simulink model "flightControlSystem"  (R2024b)
settings: Solver=ode3  StartTime=0  StopTime=10  FixedStep=Ts  RelTol=1e-3  EnableMultiTasking=on
undefined symbols (not defined in the file): codertarget, Controller, DiscIntNeverNeededParam, Discrete, Estimator, g, init, Sensors, Time, Ts, var_acc_angle_N, var_bias_gyr_N, var_gyro_p_N, Vehicle
libraries: simulink x39, sharedtransform x8, slpidlib x4, ctrlSharedLib x4, parrotlib x1
(part 3 of 3)

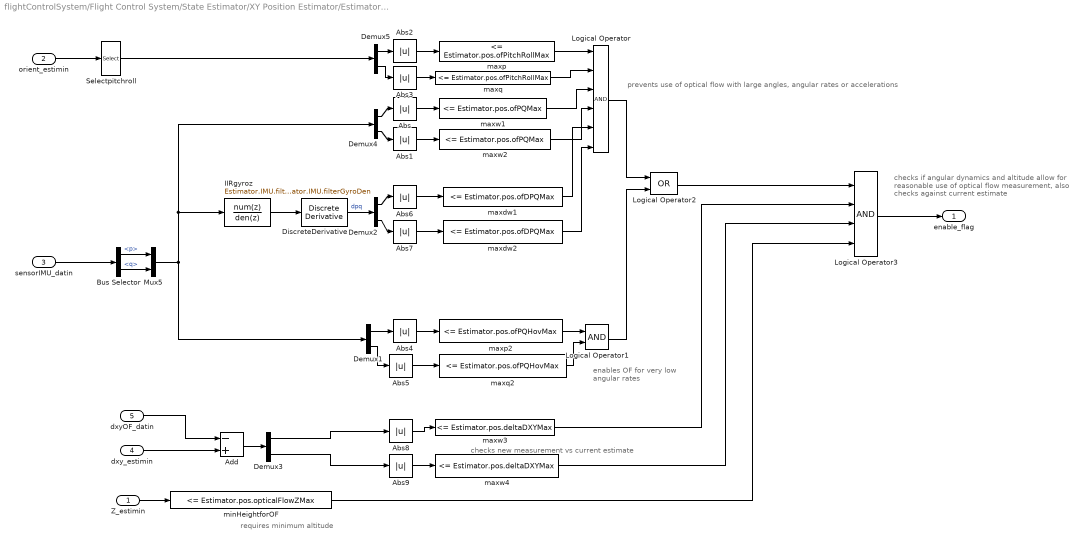
== system flightControlSystem/Flight Control System/State Estimator/XY Position Estimator/EstimatorVelocity/DataHandling ==
  note: prevents use of optical flow with large angles, angular rates or accelerations
  note: enables OF for very
      | low angular rates
  note: checks if angular dynamics and altitude allow for
      | reasonable use of optical flow measurement,
      | also checks against current estimate
  note: checks new measurement vs current estimate
  note: requires minimum altitude
  Z_estimin : Inport
  orient_estimin : Inport  Port=2
  sensorIMU_datin : Inport  Port=3
  dxy_estimin : Inport  Port=4
  dxyOF_datin : Inport  Port=5
  Abs{,1..9} (10 alike) : Abs  SaturateOnIntegerOverflow=off
  Add : Sum  Inputs=-+
  Bus Selector : BusSelector  OutputSignals=p,q
  Demux{1..5} (5 alike) : Demux  Outputs=2
  DiscreteDerivative : simulink/Discrete/Discrete Derivative  gainval=1.0  ICPrevScaledInput=0.0  OutMin=[]  OutMax=[]  OutDataType=fixdt(1, 16)  OutScaling=2^-10  DoSatur=off
  IIRgyroz : DiscreteFilter  Numerator=Estimator.IMU.filterGyroNum  Denominator=Estimator.IMU.filterGyroDen
  Logical Operator : Logic  Inputs=6  AllPortsSameDT=off  OutDataTypeStr=boolean
  Logical Operator1 : Logic  AllPortsSameDT=off  OutDataTypeStr=boolean
  Logical Operator2 : Logic  Operator=OR  AllPortsSameDT=off  OutDataTypeStr=boolean
  Logical Operator3 : Logic  Inputs=4  AllPortsSameDT=off  OutDataTypeStr=boolean
  Mux5 : Mux  Inputs=2
  Selectpitchroll : Selector  InputPortWidth=3  IndexOptions=Index vector (dialog)  Indices=[2 3]  OutputSizes=1
  maxdw1 : simulink/Logic and Bit Operations/Compare To Constant  relop=<=  const=Estimator.pos.ofDPQMax  OutDataTypeStr=boolean
  maxdw2 : simulink/Logic and Bit Operations/Compare To Constant  relop=<=  const=Estimator.pos.ofDPQMax  OutDataTypeStr=boolean
  maxp : simulink/Logic and Bit Operations/Compare To Constant  relop=<=  const=Estimator.pos.ofPitchRollMax  OutDataTypeStr=boolean
  maxp2 : simulink/Logic and Bit Operations/Compare To Constant  relop=<=  const=Estimator.pos.ofPQHovMax  OutDataTypeStr=boolean
  maxq : simulink/Logic and Bit Operations/Compare To Constant  relop=<=  const=Estimator.pos.ofPitchRollMax  OutDataTypeStr=boolean
  maxq2 : simulink/Logic and Bit Operations/Compare To Constant  relop=<=  const=Estimator.pos.ofPQHovMax  OutDataTypeStr=boolean
  maxw1 : simulink/Logic and Bit Operations/Compare To Constant  relop=<=  const=Estimator.pos.ofPQMax  OutDataTypeStr=boolean
  maxw2 : simulink/Logic and Bit Operations/Compare To Constant  relop=<=  const=Estimator.pos.ofPQMax  OutDataTypeStr=boolean
  maxw3 : simulink/Logic and Bit Operations/Compare To Constant  relop=<=  const=Estimator.pos.deltaDXYMax  OutDataTypeStr=boolean
  maxw4 : simulink/Logic and Bit Operations/Compare To Constant  relop=<=  const=Estimator.pos.deltaDXYMax  OutDataTypeStr=boolean
  minHeightforOF : simulink/Logic and Bit Operations/Compare To Constant  relop=<=  const=Estimator.pos.opticalFlowZMax  OutDataTypeStr=boolean
  enable_flag : Outport  VectorParamsAs1DForOutWhenUnconnected=off
  wires:
  minHeightforOF/1 -> Logical Operator3/4
  IIRgyroz/1 -> DiscreteDerivative/1
  Mux5/1 -> Demux1/1, Demux4/1, IIRgyroz/1
  maxw4/1 -> Logical Operator3/3
  maxw3/1 -> Logical Operator3/2
  dxyOF_datin/1 -> Add/1
  Demux3/2 -> Abs9/1
  Demux3/1 -> Abs8/1
  dxy_estimin/1 -> Add/2
  Add/1 -> Demux3/1
  Abs9/1 -> maxw4/1
  Abs8/1 -> maxw3/1
  Logical Operator2/1 -> Logical Operator3/1
  Logical Operator3/1 -> enable_flag/1
  DiscreteDerivative/1 -> Demux2/1  "dpq"
  Demux2/2 -> Abs7/1
  Demux2/1 -> Abs6/1
  Abs7/1 -> maxdw2/1
  Abs6/1 -> maxdw1/1
  Logical Operator1/1 -> Logical Operator2/2
  Demux1/2 -> Abs5/1
  Demux1/1 -> Abs4/1
  Abs5/1 -> maxq2/1
  Abs4/1 -> maxp2/1
  Abs3/1 -> maxq/1
  Abs2/1 -> maxp/1
  Demux4/2 -> Abs1/1
  Demux4/1 -> Abs/1
  Abs1/1 -> maxw2/1
  Abs/1 -> maxw1/1
  Z_estimin/1 -> minHeightforOF/1
  Logical Operator/1 -> Logical Operator2/1
  maxw1/1 -> Logical Operator/3
  Bus Selector/1 -> Mux5/1  "<p>"
  Selectpitchroll/1 -> Demux5/1
  sensorIMU_datin/1 -> Bus Selector/1
  maxq2/1 -> Logical Operator1/2
  Bus Selector/2 -> Mux5/2  "<q>"
  maxp/1 -> Logical Operator/1
  maxw2/1 -> Logical Operator/4
  orient_estimin/1 -> Selectpitchroll/1
  maxdw1/1 -> Logical Operator/5
  maxdw2/1 -> Logical Operator/6
  maxq/1 -> Logical Operator/2
  Demux5/1 -> Abs2/1
  Demux5/2 -> Abs3/1
  maxp2/1 -> Logical Operator1/1

== system flightControlSystem/Flight Control System/State Estimator/XY Position Estimator/EstimatorVelocity/XY velocity w//o angular velocity compensation ==
  note: Optical flow raw readings are converted to velocity in m/s based on the estimated altitude
  optical_flow : Inport
  z_estimate : Inport  Port=2
  " " : Product  Inputs=**
  Compare To Constant : simulink/Logic and Bit Operations/Compare To Constant  relop=<  const=200*4  OutDataTypeStr=boolean
  Counter Free-Running : simulink/Sources/Counter Free-Running  NumBits=32  tsamp=-1
  Gain : Gain  Gain=-1
  Select dxy : Selector  InputPortWidth=3  IndexOptions=Index vector (dialog)  Indices=[1 2]  OutputSizes=1
  Switch : Switch  Criteria=u2 > Threshold  SaturateOnIntegerOverflow=off  InputSameDT=off
  opticalFlowErrorCorrect : Gain  Gain=1.15
  optical_flow_dx_dy : Outport
  wires:
  Select dxy/1 -> optical_flow_dx_dy/1  "optical_flow_dx_dy"
  " "/1 -> opticalFlowErrorCorrect/1
  opticalFlowErrorCorrect/1 -> Switch/3
  Gain/1 -> " "/2
  Switch/1 -> Select dxy/1
  Counter Free-Running/1 -> Compare To Constant/1
  Compare To Constant/1 -> Switch/2
  optical_flow/1 -> " "/1, Switch/1
  z_estimate/1 -> Gain/1

== matlab function flightControlSystem/Flight Control System/State Estimator/Attitude EKF quaternion1/MATLAB Function ==
  data: P output; q output; q_prec input; P_prec input; acc input; gyro input
function [P, q] = fnc(q_prec, P_prec, acc, gyro)



wx = gyro(1);
wy = gyro(2);
wz = gyro(3);

dt= 0.0025;

noise_gyro = 0.1 ;
noise_acc = 0.1 ;

w= [wx;wy;wz];

qw_p=q_prec(1);
qx_p=q_prec(2);
qy_p=q_prec(3);
qz_p=q_prec(4);

Omega = [0,-wx,-wy,-wz;
    wx,0,wz,-wy;
    wy,-wz,0,wx;
    wz,wy,-wx,0];

if norm(w)==0 
    q=q_prec;
    P=P_prec;
else    
    % 2 option pour q_hat 
    qhat = ( cos(norm(w)*dt/2)*eye(4) + 2/norm(w)*sin(norm(w)*dt/2)*Omega)* q_prec ;
    qhat = qhat/ norm(qhat);

    % qhat = (eye(4) + dt/2*Omega)*q_prec ; 

    qhatw = qhat(1);
    qhatx = qhat(2);
    qhaty = qhat(3);
    qhatz = qhat(4);

    F=dt/2*[2/dt,-wx,-wy,-wz;
        wx,2/dt,wz,-wy;
        wy,-wz,2/dt,wx;
        wz,wy,-wx,2/dt];

    Wt = dt/2*[-qx_p,-qy_p,-qz_p;
        qw_p,-qz_p,qy_p;
        qz_p,qw_p,-qx_p;
        -qy_p,qx_p,qw_p];
    Qt = (noise_gyro^2)* (Wt)*(Wt');

    P_hat = F*P_prec*F'+Qt;

    z = [acc(1),acc(2),acc(3)]';
    z = z/norm(z);

    G= [0 ,0 ,-9.81]'; %ned ou enu ?

    C = [qhatw^2 + qhatx^2 - qhaty^2 - qhatz^2,  2*(qhatx*qhaty - qhatw*qhatz),  2*(qhatx*qhatz + qhatw*qhaty);
     2*(qhatx*qhaty + qhatw*qhatz),  qhatw^2 - qhatx^2 + qhaty^2 - qhatz^2,  2*(qhaty*qhatz - qhatw*qhatx);
     2*(qhatx*qhatz - qhatw*qhaty),  2*(qhaty*qhatz + qhatw*qhatx),  qhatw^2 - qhatx^2 - qhaty^2 + qhatz^2 ];

    h = C'*G ; 
    g = -9.81; % -0.02
    % g = -9.81  ; 
    % h= 2*[g*(qhatx*qhatz-qhatw*qhaty);
    %    g*(qhatw*qhatx+qhaty*qhatz);
    %    g*(.5-qhatx^2-qhaty^2)];

   

     h = h/norm(h);

    H = 2* [-g*qhaty, g*qhatz, -g*qhatw, g*qhatx;
       g*qhatx, g*qhatw,g*qhatz, g*qhaty;
       g*qhatw, -g*qhatx, -g*qhaty, g*qhatz];

    R = noise_acc^2 * eye(3);
    % alpha = 0.9; % Adjust this parameter between 0.9 and 1.0
    % z = alpha * z + (1 - alpha) * h;

    v = z - h ;
    S= H*P_hat*H' + R ;
    invS = inv(S);
    K=P_hat*H'*invS;
    q = qhat + K*v ;

    P = (eye(4)-K*H)*P_hat;

    q= q/norm(q);
end
    
end

== matlab function flightControlSystem/Flight Control System/Controller/Position Controller/Position error transformation (Earth to Body frame) ==
  data: yaw input; xy_err_earth input; xy_err_body output
function xy_err_body = fcn(yaw,xy_err_earth)

transformation = [cos(yaw), sin(yaw); -sin(yaw),  cos(yaw)];
xy_err_body = transformation * xy_err_earth;


end

== matlab function flightControlSystem/Flight Control System/State Estimator/Attitude EKF quaternion + yaw using basic estimator /MATLAB Function ==
  data: q output; P output; q_prec input; P_prec input; acc input; gyro input; yaw output; pitch output; roll output
function [q, P, yaw ,pitch, roll] = fnc(q_prec, P_prec, acc, gyro)



wx = gyro(1);
wy = gyro(2);
wz = gyro(3);

dt= 0.0025;

noise_gyro = 0.3 ;
noise_acc = 0.5 ;

w= [wx;wy;wz];

qw_p=q_prec(1);
qx_p=q_prec(2);
qy_p=q_prec(3);
qz_p=q_prec(4);

Omega = [0,-wx,-wy,-wz;
    wx,0,wz,-wy;
    wy,-wz,0,wx;
    wz,wy,-wx,0];

if norm(w)==0 
    q=q_prec;
    P=P_prec;
    w = q(1);
    x = q(2);
    y = q(3);
    z = q(4);
    yaw = atan2(2 * (w * z + x * y), 1 - 2 * (y^2 + z^2));
    pitch = asin(2 * (w * y - x * z));
    roll = atan2(2 * (w * x + y * z), 1 - 2 * (x^2 + y^2));


else 
    % 2 option pour q_hat 
    qhat = ( cos(norm(w)*dt/2)*eye(4) + 2/norm(w)*sin(norm(w)*dt/2)*Omega)* q_prec ;

    % qhat = (eye(4) + dt/2*Omega)*q_prec ; 

    qhatw = qhat(1);
    qhatx = qhat(2);
    qhaty = qhat(3);
    qhatz = qhat(4);

    F=dt/2*[2/dt,-wx,-wy,-wz;
        wx,2/dt,wz,-wy;
        wy,-wz,2/dt,wx;
        wz,wy,-wx,2/dt];

    Wt = dt/2*[-qx_p,-qy_p,-qz_p;
        qw_p,-qz_p,qy_p;
        qz_p,qw_p,-qx_p;
        -qy_p,qx_p,qw_p];
    Qt = (noise_gyro^2)* (Wt)*(Wt');

    P_hat = F*P_prec*F'+Qt;

    z = [acc(1),acc(2),acc(3)]';
    z = z/norm(z);

    g=-1; %ned ou enu ?

    h= 2*[g*(qhatx*qhatz-qhatw*qhaty);
       g*(qhatw*qhatx+qhaty*qhatz);
       g*(.5-qhatx^2-qhaty^2)];

    h = h/norm(h);

    H = 2* [-g*qhaty, g*qhatz, -g*qhatw, g*qhatx;
       g*qhatx, g*qhatw,g*qhatz, g*qhaty;
       g*qhatw, -g*qhatx, -g*qhaty, g*qhatz];

    R = noise_acc^2 * eye(3);

    v = z - h ;
    S= H*P_hat*H' + R ;
    invS = inv(S);
    K=P_hat*H'*invS;
    q = qhat + K*v ;

    P = (eye(4)-K*H)*P_hat;

    q= q/norm(q);

    w = q(1);
    x = q(2);
    y = q(3);
    z = q(4);

    % Compute Yaw (ψ) - Rotation around Z-axis
    yaw = atan2(2 * (w * z + x * y), 1 - 2 * (y^2 + z^2));

    % Compute Pitch (θ) - Rotation around Y-axis
    pitch = asin(2 * (w * y - x * z));  % Beware of gimbal lock if |pitch| = 90°

    % Compute Roll (φ) - Rotation around X-axis
    roll = atan2(2 * (w * x + y * z), 1 - 2 * (x^2 + y^2));
end

== matlab function flightControlSystem/Flight Control System/State Estimator/Attitude EKF quaternion2/MATLAB Function ==
  data: P output; q output; q_prec input; P_prec input; acc input; gyro input
function [P, q] = fnc(q_prec, P_prec, acc, gyro)



wx = gyro(1);
wy = gyro(2);
wz = gyro(3);

dt= 0.0025;

noise_gyro = 0.1 ;
noise_acc = 0.1 ;

w= [wx;wy;wz];

qw_p=q_prec(1);
qx_p=q_prec(2);
qy_p=q_prec(3);
qz_p=q_prec(4);

Omega = [0,-wx,-wy,-wz;
    wx,0,wz,-wy;
    wy,-wz,0,wx;
    wz,wy,-wx,0];

if norm(w)==0 
    q=q_prec;
    P=P_prec;
else    
    % 2 option pour q_hat 
    qhat = ( cos(norm(w)*dt/2)*eye(4) + 2/norm(w)*sin(norm(w)*dt/2)*Omega)* q_prec ;
    qhat = qhat/ norm(qhat);

    % qhat = (eye(4) + dt/2*Omega)*q_prec ; 

    qhatw = qhat(1);
    qhatx = qhat(2);
    qhaty = qhat(3);
    qhatz = qhat(4);

    F=dt/2*[2/dt,-wx,-wy,-wz;
        wx,2/dt,wz,-wy;
        wy,-wz,2/dt,wx;
        wz,wy,-wx,2/dt];

    Wt = dt/2*[-qx_p,-qy_p,-qz_p;
        qw_p,-qz_p,qy_p;
        qz_p,qw_p,-qx_p;
        -qy_p,qx_p,qw_p];
    Qt = (noise_gyro^2)* (Wt)*(Wt');

    P_hat = F*P_prec*F'+Qt;

    z = [acc(1),acc(2),acc(3)]';
    z = z/norm(z);

    G= [0 ,0 ,-9.81]'; %ned ou enu ?

    C = [qhatw^2 + qhatx^2 - qhaty^2 - qhatz^2,  2*(qhatx*qhaty - qhatw*qhatz),  2*(qhatx*qhatz + qhatw*qhaty);
     2*(qhatx*qhaty + qhatw*qhatz),  qhatw^2 - qhatx^2 + qhaty^2 - qhatz^2,  2*(qhaty*qhatz - qhatw*qhatx);
     2*(qhatx*qhatz - qhatw*qhaty),  2*(qhaty*qhatz + qhatw*qhatx),  qhatw^2 - qhatx^2 - qhaty^2 + qhatz^2 ];

    h = C'*G ; 
    g = -9.81; % -0.02
    % g = -9.81  ; 
    % h= 2*[g*(qhatx*qhatz-qhatw*qhaty);
    %    g*(qhatw*qhatx+qhaty*qhatz);
    %    g*(.5-qhatx^2-qhaty^2)];

   

     h = h/norm(h);

    H = 2* [-g*qhaty, g*qhatz, -g*qhatw, g*qhatx;
       g*qhatx, g*qhatw,g*qhatz, g*qhaty;
       g*qhatw, -g*qhatx, -g*qhaty, g*qhatz];

    R = noise_acc^2 * eye(3);
    % alpha = 0.9; % Adjust this parameter between 0.9 and 1.0
    % z = alpha * z + (1 - alpha) * h;

    v = z - h ;
    S= H*P_hat*H' + R ;
    invS = inv(S);
    K=P_hat*H'*invS;
    q = qhat + K*v ;

    P = (eye(4)-K*H)*P_hat;

    q= q/norm(q);
end
    
end

== matlab function flightControlSystem/Flight Control System/State Estimator/Attitude kf quaternion/MATLAB Function1 ==
  data: acc input; gyro input; prevQuat input; q output
function q = fcn(acc, gyro, prevQuat)
    
    
    kcorr = 0.002;
    
    w = norm(gyro);
    
    sigmaW = 0.5 * [0 -gyro';...
        gyro(1) 0 gyro(3) -gyro(2);...
        gyro(2) -gyro(3) 0 gyro(1);...
        gyro(3) gyro(2) -gyro(1) 0];
    
    if w==0
        qpred = prevQuat;
    else
        qpred = (eye(4)*cos(w*0.0025) + (2/w)* sigmaW * sin(w*0.0025))*prevQuat;
    end
    
    if (w < 1) && (abs(norm(acc)-9.81) < 2.9)
        
        qpred = quaternion(qpred');

        accW = rotateframe(conj(qpred),acc');
        
        accW = accW/norm(accW);
        
        epred = [0,0,-1];

        beta = acos(epred*accW');

        hB = cross(accW',epred');

        hB = hB / norm(hB);

        qcorr = quaternion([cos(kcorr*beta/2), hB'*sin(kcorr*beta/2)]);

        qpred = qcorr * qpred;

        [a,b,c,d] = qpred.parts;
        
        qpred = [a,b,c,d]';
    end
    
q =  qpred;
end

== matlab function flightControlSystem/Flight Control System/State Estimator/Madgwick Orientation Filter/MATLAB Function ==
  data: qprec input; q output; gyro input; acc input
function q = fcn(qprec, gyro, acc)

    % Time step
    dt = 0.0025;

    % Noise parameters (can be tuned)
    beta = 0.01; % Gyroscope noise 

    % Extract previous quaternion components
    qw_p = qprec(1);
    qx_p = qprec(2);
    qy_p = qprec(3);
    qz_p = qprec(4);

    % Compute quaternion derivative from gyroscope data
    w = [0, gyro(1), gyro(2), gyro(3)];
    qdotw = 0.5 * quatmultiply(qprec', w); 

    % Compute accelerometer-based correction
    f = [ 2 * (qx_p * qz_p - qw_p * qy_p) - acc(1);
          2 * (qw_p * qx_p + qy_p * qz_p) - acc(2);
          2 * (0.5 - qx_p^2 - qy_p^2) - acc(3)];

    J = [-2 * qy_p, 2 * qz_p, -2 * qw_p,  2 * qx_p;
          2 * qx_p,  2 * qw_p,  2 * qz_p,  2 * qy_p;
          0,        -4 * qx_p, -4 * qy_p,  0];

    % Compute gradient descent correction
    GradF = J' * f; 

    % Apply correction only if GradF is nonzero
    if norm(GradF) > 0
        GradF = GradF / norm(GradF); % Normalize gradient
    end

    % Update quaternion
    q = qprec + dt * (-beta * GradF + qdotw');

    % Normalize quaternion to avoid drift
    q = q / norm(q);

end

== matlab function flightControlSystem/Flight Control System/State Estimator/Mahony Orientation Filter/MATLAB Function ==
  data: gyr input; acc input; q output; q_prev input; q_int_prev input; q_int output
function [q, q_int] = mahony_filter(gyr, acc, q_prev, q_int_prev)
    % Mahony AHRS Filter for Simulink
    % Inputs:
    %   gyr       - 3x1 gyroscope readings [gx, gy, gz] in rad/s
    %   acc       - 3x1 accelerometer readings (normalized)
    %   q_prev    - 4x1 quaternion from the previous step
    %   q_int_prev- 3x1 integral correction from the previous step
    % Outputs:
    %   q         - Updated quaternion [qw, qx, qy, qz]
    %   q_int     - Updated integral correction term

    % Constants (Tunable Gains)
    dt = 0.0025;  % Time step (400 Hz)
    Kp = 2;       % Proportional gain
    Ki = 0.01;    % Integral gain

    % Ensure input quaternion is valid
    if norm(q_prev) == 0
        q_prev = [1; 0; 0; 0];  % Initialize if zero
    end
    q = q_prev;  % Copy previous quaternion

    % Normalize accelerometer data
    acc_norm = norm(acc);
    if acc_norm == 0
        q = q_prev;  % Prevent division by zero
        q_int = q_int_prev; % Keep previous integral term
        return;
    end
    acc = acc / acc_norm;

    % Estimate gravity direction from quaternion
    g = [2*(q(2)*q(4) - q(1)*q(3));  % gx
         2*(q(1)*q(2) + q(3)*q(4));  % gy
         2*(q(1)^2 + q(4)^2) - 1];   % gz

    % Compute error between measured and estimated gravity
    error = cross(g, acc);

    % Apply integral feedback if Ki > 0
    if Ki > 0
        q_int = q_int_prev + Ki * error * dt;  % Update integral term
    else
        q_int = [0; 0; 0];  % Reset integral if Ki = 0
    end

    % Compute corrected gyro data
    corrected_gyr = gyr + Kp * error + q_int;

    % Convert corrected gyro to quaternion derivative
    omega = [0; corrected_gyr];
    dq = 0.5 * quatmultiply(q', omega')';

    % Integrate quaternion derivative
    q = q_prev + dq * dt;

    % Normalize quaternion
    q = q / norm(q);
end
